simulink model "MtrCtrl_24V"  (R2023b)
settings: Solver=FixedStepDiscrete  StartTime=0.0  StopTime=1  FixedStep=1e-6  RelTol=1e-3
values from neighbouring files (symbols this model uses):
  B = 0.001889    [MtrCtrl_v01.sldd]    (also in PICal.m = 0.001889; PMSM.m = Simulink.Parameter)
  C_LUT_AngleTable_sng_Null = saveVarsMat.C_LUT_AngleTable_sng_Null    [AngleTable.m]    (also in MtrCtrl_v01.sldd = 0.0015339807878856412 0.0030679615757712823 0.00460194236365; PMSM.m; SinLut.m = sinTable(2,:))
  C_LUT_SinTable_sng_Null = saveVarsMat.C_LUT_SinTable_sng_Null    [AngleTable.m]    (also in MtrCtrl_v01.sldd = 0.0015339801862847655 0.0030679567629659761 0.00460192612044; PMSM.m; SinLut.m = sinTable(1,:))
  C_MATH_OneOverSqrtThree_s32n31_Null = 0.57735026918962584    [MtrCtrl_v01.sldd]    (also in PMSM.m = Simulink.Parameter)
  C_MATH_Pi_u32n30_Null = 3.1415926535897931    [MtrCtrl_v01.sldd]    (also in PMSM.m = Simulink.Parameter)
  C_MATH_SqrtThreeOverThree_s32n31_Null = 0.57735026918962573    [MtrCtrl_v01.sldd]    (also in PMSM.m = Simulink.Parameter)
  C_PMSM_CurQKi_u32n31_null = 0.15707963267949    [MtrCtrl_v01.sldd]    (also in PMSM.m = Simulink.Parameter)
  C_PMSM_CurQKp_u32n31_null = 19.949113350295185    [MtrCtrl_v01.sldd]    (also in PMSM.m = Simulink.Parameter)
  C_PMSM_Flux_u32n32_Vs = 0.192    [MtrCtrl_v01.sldd]    (also in PMSM.m = Simulink.Parameter)
  C_PMSM_Ls_pu = 0.398982267005904    [MtrCtrl_v01.sldd]
  C_PMSM_PolePairs_u8_Null = 4.0    [MtrCtrl_v01.sldd]
  Flux = 0.192    [MtrCtrl_v01.sldd]    (also in PICal.m; PMSM.m)
  IBase_A = 2000.0    [MtrCtrl_v01.sldd]    (also in PICal.m = 300; PMSM.m = Simulink.Parameter)
  J = 0.011    [MtrCtrl_v01.sldd]    (also in PICal.m; PMSM.m)
  K_CCM_MRASEna_bool_Flg = 0.0    [MtrCtrl_v01.sldd]
  K_SVM_DefultDuty_s32n31_Null = 0.25    [MtrCtrl_v01.sldd]    (also in PMSM.m = Simulink.Parameter)
  KCCM_VirPosn_flg = 0.0    [MtrCtrl_v01.sldd]    (also in PMSM.m = Simulink.Parameter)
  KCCM_VoltModeEna_Flg = 0.0    [MtrCtrl_v01.sldd]    (also in PMSM.m = Simulink.Parameter)
  Kis = 114583.3333333333    [MtrCtrl_v01.sldd]    (also in PICal.m = 114583.333333; PMSM.m = 114583.333333)
  KSMO_EnaEst_Flg = 0.0    [MtrCtrl_v01.sldd]    (also in PMSM.m = Simulink.Parameter)
  Kt = 1.1520000000000001    [MtrCtrl_v01.sldd]    (also in PICal.m = 1.152; PMSM.m = 1.152)
  Ld = 80e-6    (= 8e-05)    [FluxweakingGen.m]    (also in IEHB_MAPGenerationtest.m = 6.8e-05; MtrCtrl_v01.sldd = 0.000635
                
                    
             ; PICal.m = 0.000635; PMSM.m = Simulink.Parameter)
  LPF_coefg = 0.01    [MtrCtrl_v01.sldd]    (also in PMSM.m = Simulink.Parameter)
  Lq = 80e-6    (= 8e-05)    [FluxweakingGen.m]    (also in IEHB_MAPGenerationtest.m = 6e-05; MtrCtrl_v01.sldd = 0.000685
                
                    
             ; PICal.m = 0.000635; PMSM.m = Simulink.Parameter)
  Ls = 0.000635    [MtrCtrl_v01.sldd]    (also in PICal.m; PMSM.m)
  OneOverUBase_V = 0.0016666666666666668    [MtrCtrl_v01.sldd]    (also in PMSM.m = Simulink.Parameter)
  Pp = 4.0    [MtrCtrl_v01.sldd]    (also in PICal.m = 4; PMSM.m = Simulink.Parameter)
  Rs = 0.03    [FluxweakingGen.m]    (also in MtrCtrl_v01.sldd = 0.05
                
                    
                 ; PICal.m = 0.05; PMSM.m = Simulink.Parameter)
  SecPerRnd = 0.6    [MtrCtrl_v01.sldd]    (also in PMSM.m = Simulink.Parameter)
  sinTable = zeros(2,TableSize)    [SinLut.m]
  SMOGain_V = 323.31615074619043    [MtrCtrl_v01.sldd]    (also in PMSM.m = Simulink.Parameter)
  Ts = 1.0E-6    [MtrCtrl_v01.sldd]    (also in PICal.m = 0.0001; PMSM.m = Simulink.Parameter)
  TsCtrl = 1.0E-6    [MtrCtrl_v01.sldd]
  UBase_V = 600.0    [MtrCtrl_v01.sldd]    (also in PICal.m = 600; PMSM.m = Simulink.Parameter)
  wmBase_rps = 314.15926535897933    [MtrCtrl_v01.sldd]    (also in PICal.m = 314.159265359; PMSM.m = Simulink.Parameter)
undefined symbols (not defined in the file or in its folder): DiscIntNeverNeededParam, Ion, Lithium
libraries: ee_lib x16, spsVoltageMeasurementLib x14, simulink x11, spsSeriesRLCBranchLib x6, spsMosfetLib x6, nesl_utility x6, slpidlib x5, spsCurrentMeasurementLib x4, spsParallelRLCBranchLib x3, simulink_extras x2, spspowerguiLib x2, eePmsmFwController x1
(part 4 of 5)

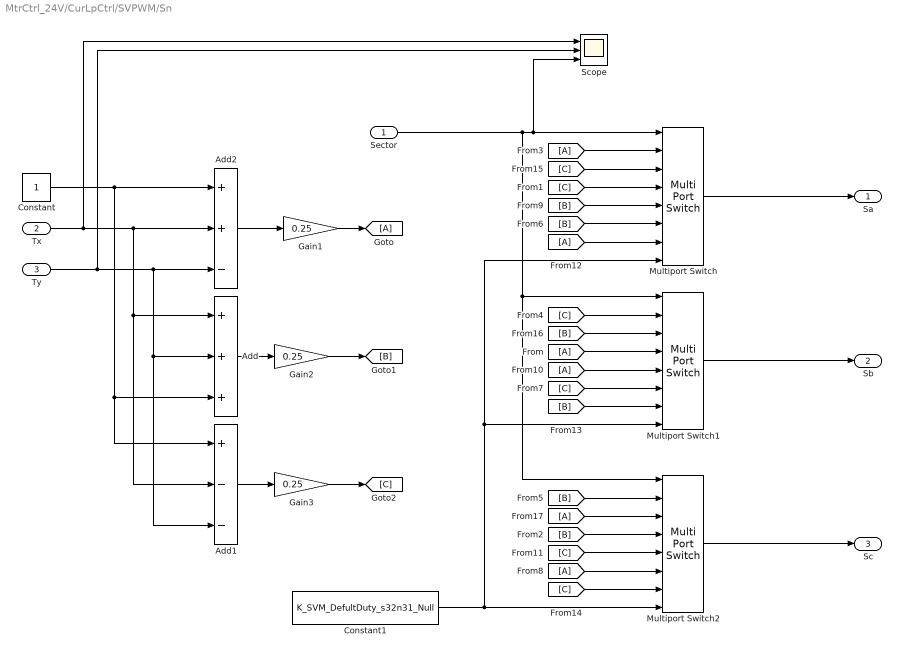
== system MtrCtrl_24V/CurLpCtrl/SVPWM/Sn ==
  Sector : Inport  OutDataTypeStr=uint8
  Tx : Inport  Port=2  OutDataTypeStr=fixdt(0,32,33)
  Ty : Inport  Port=3  OutDataTypeStr=fixdt(0,32,33)
  Add : Sum  Inputs=+++  OutDataTypeStr=fixdt(0,32,31)
  Add1 : Sum  Inputs=+--  OutDataTypeStr=fixdt(0,32,31)
  Add2 : Sum  Inputs=++-  OutDataTypeStr=fixdt(0,32,31)
  Constant : Constant  OutDataTypeStr=fixdt(0,32,31)
  Constant1 : Constant  Value=K_SVM_DefultDuty_s32n31_Null
  From{,3,8,10,12,17} (6 alike) : From
  Gain1 : Gain  Gain=0.25  OutDataTypeStr=fixdt(0,32,33)
  Gain2 : Gain  Gain=0.25  OutDataTypeStr=fixdt(0,32,33)
  Gain3 : Gain  Gain=0.25  OutDataTypeStr=fixdt(0,32,33)
  Goto : Goto
  Multiport Switch : MultiPortSwitch  Inputs=6  DataPortForDefault=Additional data port  OutDataTypeStr=fixdt(0,32,33)  SaturateOnIntegerOverflow=off  InputSameDT=off
  Multiport Switch1 : MultiPortSwitch  Inputs=6  DataPortForDefault=Additional data port  OutDataTypeStr=fixdt(0,32,33)  SaturateOnIntegerOverflow=off  InputSameDT=off
  Multiport Switch2 : MultiPortSwitch  Inputs=6  DataPortForDefault=Additional data port  OutDataTypeStr=fixdt(0,32,33)  SaturateOnIntegerOverflow=off  InputSameDT=off
  Scope : Scope  NumInputPorts=3
  Sa : Outport
  Sb : Outport  Port=2
  Sc : Outport  Port=3
  wires:
  Tx/1 -> Scope/1, Add1/2, Add/1, Add2/2
  Ty/1 -> Scope/2, Add1/3, Add/2, Add2/3
  Add/1 -> Gain2/1
  Constant/1 -> Add1/1, Add/3, Add2/1
  Add2/1 -> Gain1/1
  Add1/1 -> Gain3/1
  Sector/1 -> Multiport Switch/1, Scope/3, Multiport Switch2/1, Multiport Switch1/1
  Multiport Switch/1 -> Sa/1
  Multiport Switch1/1 -> Sb/1
  Multiport Switch2/1 -> Sc/1
  Gain1/1 -> Goto/1
  Gain2/1 -> [B]
  Gain3/1 -> [C]
  [C] -> Multiport Switch/4
  From/1 -> Multiport Switch1/4
  [B] -> Multiport Switch2/4
  From3/1 -> Multiport Switch/2
  [C] -> Multiport Switch1/2
  [B] -> Multiport Switch2/2
  [B] -> Multiport Switch/6
  [C] -> Multiport Switch1/6
  From8/1 -> Multiport Switch2/6
  [B] -> Multiport Switch/5
  From10/1 -> Multiport Switch1/5
  [C] -> Multiport Switch2/5
  From12/1 -> Multiport Switch/7
  [B] -> Multiport Switch1/7
  [C] -> Multiport Switch2/7
  [C] -> Multiport Switch/3
  [B] -> Multiport Switch1/3
  From17/1 -> Multiport Switch2/3
  Constant1/1 -> Multiport Switch/8, Multiport Switch1/8, Multiport Switch2/8

== system MtrCtrl_24V/CurLpCtrl/SVPWM/SwitchTimeCalculation ==
  N : Inport  OutDataTypeStr=fixdt(0,32,29)
  V1 : Inport  Port=2  OutDataTypeStr=fixdt(1,32,31)
  V2 : Inport  Port=3  OutDataTypeStr=fixdt(1,32,32)
  V3 : Inport  Port=4  OutDataTypeStr=fixdt(1,32,32)
  A : MultiPortSwitch  Inputs=6  OutDataTypeStr=fixdt(1,32,32)  SaturateOnIntegerOverflow=off  InputSameDT=off
  B : MultiPortSwitch  Inputs=6  OutDataTypeStr=fixdt(1,32,31)  SaturateOnIntegerOverflow=off  InputSameDT=off
  C : MultiPortSwitch  Inputs=6  OutDataTypeStr=fixdt(1,32,31)  SaturateOnIntegerOverflow=off  InputSameDT=off
  Gain1 : Gain  Gain=-1  ParamDataTypeStr=fixdt(1,32,31)  OutDataTypeStr=fixdt(1,32,32)
  Gain2 : Gain  Gain=-1  ParamDataTypeStr=fixdt(1,32,31)  OutDataTypeStr=fixdt(1,32,31)
  Gain3 : Gain  Gain=-1  ParamDataTypeStr=fixdt(1,32,31)  OutDataTypeStr=fixdt(1,32,32)
  Sum : Sum  Inputs=|++  OutDataTypeStr=fixdt(1,32,32)  AccumDataTypeStr=fixdt(1,32,32)
  Sum1 : Sum  Inputs=-+|  OutDataTypeStr=fixdt(1,32,30)  AccumDataTypeStr=fixdt(1,32,30)
  Sum2 : Sum  Inputs=|++  OutDataTypeStr=fixdt(1,32,30)  AccumDataTypeStr=fixdt(1,32,30)
  Ta : Outport
  Tb : Outport  Port=2
  Tc : Outport  Port=3
  wires:
  N/1 -> A/1, B/1, C/1
  A/1 -> Ta/1
  B/1 -> Tb/1
  C/1 -> Tc/1
  V2/1 -> Gain1/1, A/2, A/5, Sum/1
  V3/1 -> Gain3/1, A/7, A/4, Sum/2, Sum1/1
  Sum/1 -> A/6, A/3
  V1/1 -> Gain2/1, B/3, B/6, Sum1/2
  Sum1/1 -> B/2, B/5
  Gain3/1 -> B/4, B/7
  Gain1/1 -> C/5, C/2, Sum2/1
  Gain2/1 -> C/3, C/6, Sum2/2
  Sum2/1 -> C/7, C/4

== system MtrCtrl_24V/CurLpCtrl/SVPWM/TempValueCalculation ==
  V_alpha : Inport  OutDataTypeStr=fixdt(1,32,31)
  V_beta : Inport  Port=2  OutDataTypeStr=fixdt(1,32,31)
  Add : Sum  Inputs=+-  OutDataTypeStr=fixdt(1,32,32)
  Add1 : Sum  OutDataTypeStr=fixdt(1,32,32)
  Gain : Gain  Gain=0.5  OutDataTypeStr=fixdt(1,32,32)
  Gain1 : Gain  Gain=sqrt(3)/2  OutDataTypeStr=fixdt(1,32,33)
  V1 : Outport  VectorParamsAs1DForOutWhenUnconnected=off
  V2 : Outport  Port=2  VectorParamsAs1DForOutWhenUnconnected=off
  V3 : Outport  Port=3  VectorParamsAs1DForOutWhenUnconnected=off
  wires:
  V_alpha/1 -> Gain1/1
  Gain1/1 -> Add1/2
  Add1/1 -> V2/1, Add/1  "V2"
  V_beta/1 -> Gain/1, Add/2, V1/1  "V1"
  Add/1 -> V3/1  "V3"
  Gain/1 -> Add1/1

== system MtrCtrl_24V/CurLpCtrl/Subsystem10/Subsystem ==
  idqRef : Inport  OutDataTypeStr=fixdt(1,32,31)
  vdq : Inport  Port=2  OutDataTypeStr=fixdt(1,32,31)
  VphMax : Inport  Port=3  OutDataTypeStr=fixdt(0,32,32)
  Cartesian to Polar : Subsystem  Tag=DecoupledSystem
  Constant : Constant  Value=C_MATH_Pi_u32n30_Null  OutDataTypeStr=fixdt(0,32,30)  SampleTime=-1
  Demux : Demux  Outputs=2
  Discrete-Time Integrator : DiscreteIntegrator  IntegratorMethod=Integration: Backward Euler  gainval=5  InitialCondition=1  SampleTime=-1  OutDataTypeStr=fixdt(1,32,28)  ICPrevOutput=DiscIntNeverNeededParam  ICPrevScaledInput=DiscIntNeverNeededParam
  Gain : Gain  Gain=50  OutDataTypeStr=fixdt(1,32,25)
  Gain1 : Gain  Gain=10  OutDataTypeStr=fixdt(1,32,25)
  Gain2 : Gain  Gain=2
  Modulation index threshold : Constant  Value=C_MATH_SqrtThreeOverThree_s32n31_Null  OutDataTypeStr=fixdt(0,32,31)  SampleTime=-1
  Modulation index threshold1 : Constant  Value=3.24  OutDataTypeStr=fixdt(0,32,30)  SampleTime=-1
  Mux : Mux  Inputs=2
  Polar to Cartesian : Subsystem  Tag=DecoupledSystem
  Product : Product  OutDataTypeStr=fixdt(1,32,28)
  Saturation : Saturate  UpperLimit=1  LowerLimit=0  OutDataTypeStr=fixdt(1,32,28)
  Subsystem1 : Subsystem
  Sum : Sum  Inputs=|-+  OutDataTypeStr=fixdt(1,32,30)
  Sum1 : Sum  Inputs=|-+  OutDataTypeStr=fixdt(1,32,28)
  Sum2 : Sum  Inputs=|-+  OutDataTypeStr=fixdt(1,32,28)
  Sum3 : Sum  Inputs=-+  OutDataTypeStr=fixdt(1,32,28)
  Sum4 : Sum  Inputs=|++  OutDataTypeStr=fixdt(1,32,25)
  Unit Delay : UnitDelay  SampleTime=-1  HasFrameUpgradeWarning=on
  idqRefFW : Outport  VectorParamsAs1DForOutWhenUnconnected=off
  wires:
  Product/1 -> Sum2/1
  Sum1/1 -> Product/1
  Gain1/1 -> Sum4/2
  Cartesian to Polar/1(Out1) -> Polar to Cartesian/1(In1)
  Subsystem1/1(M) -> Sum/1
  Sum/1 -> Gain/1
  Discrete-Time Integrator/1 -> Saturation/1, Sum3/1
  Unit Delay/1 -> Gain1/1
  Cartesian to Polar/2(Out2) -> Sum1/1
  Polar to Cartesian/2(Out2) -> Mux/2
  Mux/1 -> idqRefFW/1
  Gain/1 -> Sum4/1
  VphMax/1 -> Subsystem1/2(VphMax)
  Modulation index threshold/1 -> Gain2/1
  Saturation/1 -> Product/2, Sum3/2
  Demux/2 -> Cartesian to Polar/2(In2)
  Demux/1 -> Cartesian to Polar/1(In1)
  idqRef/1 -> Demux/1
  Polar to Cartesian/1(Out1) -> Mux/1
  Constant/1 -> Sum1/2, Sum2/2
  Sum3/1 -> Unit Delay/1
  vdq/1 -> Subsystem1/1(vdq)
  Sum2/1 -> Polar to Cartesian/2(In2)
  Sum4/1 -> Discrete-Time Integrator/1
  Gain2/1 -> Sum/2

== system MtrCtrl_24V/CurLpCtrl/Subsystem2/Subsystem1 ==
  In1 : Inport  OutDataTypeStr=fixdt(0,32,0)
  Constant7 : Constant  Value=2*pi  OutDataTypeStr=fixdt(0,32,0)
  Mod : Math  Operator=mod
  Out1 : Outport
  wires:
  Mod/1 -> Out1/1
  In1/1 -> Mod/1
  Constant7/1 -> Mod/2

== system MtrCtrl_24V/CurLpCtrl/Subsystem2/Subsystem2 ==
  FilterIn : Inport  OutDataTypeStr=fixdt(1,32,31)
  Rest : Inport  Port=2  OutDataTypeStr=fixdt(1,32,0)
  Add : Sum  Inputs=+-  OutDataTypeStr=fixdt(1,32,31)
  Add1 : Sum  OutDataTypeStr=fixdt(1,32,31)
  Constant : Constant  Value=LPF_coefg  OutDataTypeStr=fixdt(0,32,31)
  Delay : Delay  DelayLength=1  ExternalReset=Either
      settings: InputPortMap=u0,r5
  Product : Product  OutDataTypeStr=fixdt(1,32,31)
  FilterOut : Outport
  wires:
  FilterIn/1 -> Add/1
  Add/1 -> Product/2
  Product/1 -> Add1/1
  Add1/1 -> Delay/1, FilterOut/1
  Delay/1 -> Add/2, Add1/2
  Rest/1 -> Delay/2
  Constant/1 -> Product/1

== system MtrCtrl_24V/CurLpCtrl/Subsystem2/Subsystem3 ==
  ParkPosn : Inport  OutDataTypeStr=fixdt(1,32,28)
  1-D Lookup Table : Lookup_n-D  NumberOfTableDimensions=1  BreakpointsForDimension1=sinTable(2,:)  BeginIndexSearchUsingPreviousIndexResult=on  Table=sinTable(1,:)  ExtrapMethod=Clip  UseLastTableValue=on  ApplyFullPrecisionForLinearInterpolation=on  InternalRulePriority=Speed  OutDataTypeStr=fixdt(0,32,31)  RndMeth=Simplest
  1-D Lookup Table1 : Lookup_n-D  NumberOfTableDimensions=1  BreakpointsForDimension1=sinTable(2,:)  BeginIndexSearchUsingPreviousIndexResult=on  Table=sinTable(1,:)  ExtrapMethod=Clip  UseLastTableValue=on  ApplyFullPrecisionForLinearInterpolation=on  InternalRulePriority=Speed  OutDataTypeStr=fixdt(0,32,31)  RndMeth=Simplest
  Add : Sum  OutDataTypeStr=fixdt(1,32,26)
  Chart : Stateflow chart  TreatAsAtomicUnit=on
  Constant1 : Constant  Value=0  OutDataTypeStr=fixdt(1,32,4)
  Gain : Gain  Gain=4  OutDataTypeStr=fixdt(1,32,26)
  Product : Product  OutDataTypeStr=fixdt(1,32,30)  RndMeth=Simplest
  Product1 : Product  OutDataTypeStr=fixdt(1,32,30)
  Scope : Scope  NumInputPorts=3
  SinTheta : Outport
  CosTheta : Outport  Port=2
  wires:
  ParkPosn/1 -> Gain/1
  Gain/1 -> Add/2
  Constant1/1 -> Add/1
  Product/1 -> Scope/1, SinTheta/1
  Product1/1 -> Scope/2, CosTheta/1
  Add/1 -> Scope/3, Chart/1(Angle)
  Chart/1(SinAngle) -> 1-D Lookup Table/1
  Chart/3(CosAngle) -> 1-D Lookup Table1/1
  1-D Lookup Table/1 -> Product/1
  Chart/2(SinSign) -> Product/2
  1-D Lookup Table1/1 -> Product1/1
  Chart/4(CosSign) -> Product1/2

== system MtrCtrl_24V/CurLpCtrl/Subsystem2/Subsystem4 ==
  FilterIn : Inport  OutDataTypeStr=fixdt(1,32,31)
  Rest : Inport  Port=2  OutDataTypeStr=fixdt(1,32,0)
  Add : Sum  Inputs=+-  OutDataTypeStr=fixdt(1,32,31)
  Add1 : Sum  OutDataTypeStr=fixdt(1,32,31)
  Constant : Constant  Value=LPF_coefg  OutDataTypeStr=fixdt(0,32,31)
  Delay : Delay  DelayLength=1  ExternalReset=Either
      settings: InputPortMap=u0,r5
  Product : Product  OutDataTypeStr=fixdt(1,32,31)
  FilterOut : Outport
  wires:
  Rest/1 -> Delay/2
  Delay/1 -> Add1/2, Add/2
  Add1/1 -> FilterOut/1, Delay/1
  Product/1 -> Add1/1
  Add/1 -> Product/2
  FilterIn/1 -> Add/1
  Constant/1 -> Product/1

== system MtrCtrl_24V/CurLpCtrl/Subsystem2/Subsystem5 ==
  FilterIn : Inport  OutDataTypeStr=fixdt(1,32,22)
  Rest : Inport  Port=2  OutDataTypeStr=fixdt(1,32,0)
  Add : Sum  Inputs=+-  OutDataTypeStr=fixdt(1,32,23)
  Add1 : Sum  OutDataTypeStr=fixdt(1,32,22)
  Constant : Constant  Value=LPF_coefg  OutDataTypeStr=fixdt(0,32,38)
  Delay : Delay  DelayLength=1  ExternalReset=Either
      settings: InputPortMap=u0,r5
  Product : Product  OutDataTypeStr=fixdt(1,32,29)
  FilterOut : Outport
  wires:
  FilterIn/1 -> Add/1
  Add/1 -> Product/2
  Product/1 -> Add1/1
  Add1/1 -> Delay/1, FilterOut/1
  Delay/1 -> Add/2, Add1/2
  Rest/1 -> Delay/2
  Constant/1 -> Product/1

== system MtrCtrl_24V/CurLpCtrl/Subsystem2/Z_alpha ==
  Salpha : Inport  OutDataTypeStr=int32
  Constant : Constant  OutDataTypeStr=fixdt(1,32,30)
  Constant1 : Constant  Value=-1  OutDataTypeStr=fixdt(1,32,30)
  Divide : Product  Inputs=*/  OutDataTypeStr=fixdt(1,32,30)
  E : Constant  Value=600  OutDataTypeStr=int32
  If : If  NumInputs=2  IfExpression=u1 > u2  ElseIfExpressions=u1 < -u2
  If Action Subsystem : Subsystem  TreatAsAtomicUnit=on
  If Action Subsystem1 : Subsystem  TreatAsAtomicUnit=on
  If Action Subsystem2 : Subsystem  TreatAsAtomicUnit=on
  Merge : Merge  Inputs=3
  ZalphaOut : Outport
  wires:
  Salpha/1 -> If/1, Divide/1
  E/1 -> If/2, Divide/2
  Divide/1 -> If Action Subsystem2/1(In1)
  If/1 -> If Action Subsystem/Action
  If Action Subsystem/1(ZalphaOut) -> Merge/1
  If/3 -> If Action Subsystem2/Action
  If/2 -> If Action Subsystem1/Action
  If Action Subsystem1/1(ZalphaOut) -> Merge/2
  If Action Subsystem2/1(ZalphaOut) -> Merge/3
  Merge/1 -> ZalphaOut/1
  Constant/1 -> If Action Subsystem/1(In1)
  Constant1/1 -> If Action Subsystem1/1(In1)

== system MtrCtrl_24V/CurLpCtrl/Subsystem2/Z_alpha1 ==
  Salpha : Inport  OutDataTypeStr=int32
  Constant : Constant  OutDataTypeStr=fixdt(1,32,30)
  Constant1 : Constant  Value=-1  OutDataTypeStr=fixdt(1,32,30)
  Divide : Product  Inputs=*/  OutDataTypeStr=fixdt(1,32,30)
  E : Constant  Value=600  OutDataTypeStr=int32
  If : If  NumInputs=2  IfExpression=u1 > u2  ElseIfExpressions=u1 < -u2
  If Action Subsystem : Subsystem  TreatAsAtomicUnit=on
  If Action Subsystem1 : Subsystem  TreatAsAtomicUnit=on
  If Action Subsystem2 : Subsystem  TreatAsAtomicUnit=on
  Merge : Merge  Inputs=3
  ZalphaOut : Outport
  wires:
  Constant1/1 -> If Action Subsystem1/1(In1)
  Constant/1 -> If Action Subsystem/1(In1)
  Merge/1 -> ZalphaOut/1
  If Action Subsystem2/1(ZalphaOut) -> Merge/3
  If Action Subsystem1/1(ZalphaOut) -> Merge/2
  If/2 -> If Action Subsystem1/Action
  If/3 -> If Action Subsystem2/Action
  If Action Subsystem/1(ZalphaOut) -> Merge/1
  If/1 -> If Action Subsystem/Action
  Divide/1 -> If Action Subsystem2/1(In1)
  E/1 -> Divide/2, If/2
  Salpha/1 -> Divide/1, If/1

== system MtrCtrl_24V/CurLpCtrl/Subsystem4/SinCos ==
  In1 : Inport  LockScale=on
  DTC_input_1 : DataTypeConversion  OutDataTypeStr=fixdt('double')  RndMeth=Nearest  SaturateOnIntegerOverflow=off  LockScale=on
  DTC_output_1 : DataTypeConversion  OutDataTypeStr=fixdt(1,32,4)  SaturateOnIntegerOverflow=off  RndMeth=Floor
  DTC_output_2 : DataTypeConversion  OutDataTypeStr=fixdt(0,32,31)  SaturateOnIntegerOverflow=off  RndMeth=Floor
  ReplicaOfSource : Trigonometry  Operator=sincos
  Out1 : Outport  LockScale=on
  Out2 : Outport  Port=2  LockScale=on
  wires:
  In1/1 -> DTC_input_1/1
  DTC_output_1/1 -> Out1/1
  ReplicaOfSource/1 -> DTC_output_1/1
  ReplicaOfSource/2 -> DTC_output_2/1
  DTC_input_1/1 -> ReplicaOfSource/1
  DTC_output_2/1 -> Out2/1

== system MtrCtrl_24V/CurLpCtrl/Subsystem8/Subsystem ==
  Id_k : Inport
  Iq_k : Inport  Port=2
  we_k : Inport  Port=3
  Ud_k : Inport  Port=4
  Uq_k : Inport  Port=5
  Add2 : Sum
  Add3 : Sum
  Add4 : Sum
  Add5 : Sum  Inputs=+++
  Constant1 : Constant  Value=1-TsCtrl*Rs/Ls
  Constant18 : Constant  Value=-TsCtrl*Flux/Ls
  Constant2 : Constant  Value=TsCtrl/Ls
  Constant3 : Constant  Value=1-TsCtrl*Rs/Ls
  Constant4 : Constant  Value=TsCtrl/Ls
  Gain6 : Gain  Gain=TsCtrl
  Gain7 : Gain  Gain=-1
  Id_k_copy : InportShadow
  Iq_k_copy : InportShadow  Port=2
  Product{5,9..14} (7 alike) : Product
  Subtract : Sum  Inputs=+-
  Subtract1 : Sum  Inputs=+-
  Dlt_Id : Outport
  Dlt_Iq : Outport  Port=2
  wires:
  Product14/1 -> Add5/3
  Constant2/1 -> Product13/1
  Product10/1 -> Add3/1
  Gain6/1 -> Gain7/1, Product9/2
  Constant1/1 -> Product11/1
  Uq_k/1 -> Product13/2
  Product5/1 -> Add2/1
  Product9/1 -> Add2/2
  Product12/1 -> Add4/2
  Id_k/1 -> Product10/2, Product5/1
  Product11/1 -> Add3/2
  Constant4/1 -> Product12/1
  Add2/1 -> Add4/1
  Iq_k/1 -> Product11/2, Product9/1
  Constant18/1 -> Product14/1
  Add5/1 -> Subtract1/1  "Iq_k_1"
  we_k/1 -> Product14/2, Gain6/1
  Gain7/1 -> Product10/1
  Constant3/1 -> Product5/2
  Add3/1 -> Add5/1
  Add4/1 -> Subtract/1  "Id_k_1"
  Product13/1 -> Add5/2
  Ud_k/1 -> Product12/2
  Id_k_copy/1 -> Subtract/2
  Subtract/1 -> Dlt_Id/1
  Subtract1/1 -> Dlt_Iq/1
  Iq_k_copy/1 -> Subtract1/2

== system MtrCtrl_24V/CurLpCtrl/Subsystem8/Subsystem3 ==
  Id_k1 : Inport
  Iq_k1 : Inport  Port=2
  we_k : Inport  Port=3
  Ud_k1 : Inport  Port=4
  Uq_k1 : Inport  Port=5
  Add2 : Sum
  Add3 : Sum
  Add4 : Sum
  Add5 : Sum  Inputs=+++
  Constant1 : Constant  Value=1-Ts*Rs/Ls
  Constant14 : Constant  Value=1-Ts*Rs/Ls
  Constant16 : Constant  Value=Ts/Ls
  Constant18 : Constant  Value=-Ts*Flux/Ls
  Constant2 : Constant  Value=Ts/Ls
  Gain6 : Gain  Gain=TsCtrl
  Gain7 : Gain  Gain=-1
  Id_k1_Copy : InportShadow
  Iq_k1_Copy : InportShadow  Port=2
  Product{5,9..14} (7 alike) : Product
  Subtract : Sum  Inputs=+-
  Subtract1 : Sum  Inputs=+-
  Dlt_Id : Outport
  Dlt_Iq : Outport  Port=2
  wires:
  Iq_k1_Copy/1 -> Subtract1/2
  Subtract1/1 -> Dlt_Iq/1
  Subtract/1 -> Dlt_Id/1
  Id_k1_Copy/1 -> Subtract/2
  Ud_k1/1 -> Product12/2
  Product13/1 -> Add5/2
  Add4/1 -> Subtract/1  "Id_k2"
  Add3/1 -> Add5/1
  Constant14/1 -> Product5/2
  Gain7/1 -> Product10/1
  we_k/1 -> Gain6/1, Product14/2
  Add5/1 -> Subtract1/1  "Iq_k2"
  Constant18/1 -> Product14/1
  Iq_k1/1 -> Product9/1, Product11/2
  Add2/1 -> Add4/1
  Constant16/1 -> Product12/1
  Product11/1 -> Add3/2
  Id_k1/1 -> Product5/1, Product10/2
  Product12/1 -> Add4/2
  Product9/1 -> Add2/2
  Product5/1 -> Add2/1
  Uq_k1/1 -> Product13/2
  Constant1/1 -> Product11/1
  Gain6/1 -> Product9/2, Gain7/1
  Product10/1 -> Add3/1
  Constant2/1 -> Product13/1
  Product14/1 -> Add5/3

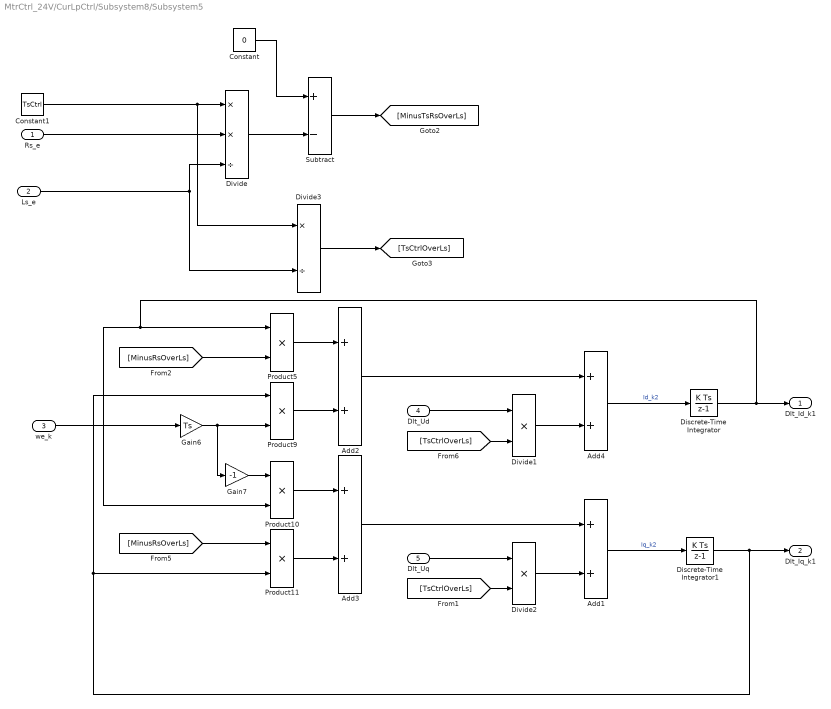
== system MtrCtrl_24V/CurLpCtrl/Subsystem8/Subsystem5 ==
  Rs_e : Inport
  Ls_e : Inport  Port=2
  we_k : Inport  Port=3
  Dlt_Ud : Inport  Port=4
  Dlt_Uq : Inport  Port=5
  Add{1..4} (4 alike) : Sum
  Constant : Constant  Value=0
  Constant1 : Constant  Value=TsCtrl
  Discrete-Time Integrator : DiscreteIntegrator  SampleTime=-1  ICPrevOutput=DiscIntNeverNeededParam  ICPrevScaledInput=DiscIntNeverNeededParam
  Discrete-Time Integrator1 : DiscreteIntegrator  SampleTime=-1  ICPrevOutput=DiscIntNeverNeededParam  ICPrevScaledInput=DiscIntNeverNeededParam
  Divide : Product  Inputs=**/
  Divide1 : Product  Inputs=**
  Divide2 : Product  Inputs=**
  Divide3 : Product  Inputs=*/
  Gain6 : Gain  Gain=Ts
  Gain7 : Gain  Gain=-1
  Product{5,9..11} (4 alike) : Product
  Subtract : Sum  Inputs=+-
  Dlt_Id_k1 : Outport
  Dlt_Iq_k1 : Outport  Port=2
  wires:
  Dlt_Ud/1 -> Divide1/1
  Divide2/1 -> Add1/2
  Add4/1 -> Discrete-Time Integrator/1  "Id_k2"
  Add3/1 -> Add1/1
  [MinusRsOverLs] -> Product5/2
  Gain7/1 -> Product10/1
  we_k/1 -> Gain6/1
  Add1/1 -> Discrete-Time Integrator1/1  "Iq_k2"
  Discrete-Time Integrator1/1 -> Dlt_Iq_k1/1, Product9/1, Product11/2
  Add2/1 -> Add4/1
  [TsCtrlOverLs] -> Divide1/2
  Product11/1 -> Add3/2
  Discrete-Time Integrator/1 -> Product10/2, Product5/1, Dlt_Id_k1/1
  Divide1/1 -> Add4/2
  Product9/1 -> Add2/2
  Product5/1 -> Add2/1
  Dlt_Uq/1 -> Divide2/1
  [MinusRsOverLs] -> Product11/1
  Gain6/1 -> Product9/2, Gain7/1
  Product10/1 -> Add3/1
  Constant/1 -> Subtract/1
  Rs_e/1 -> Divide/2
  Divide/1 -> Subtract/2
  Subtract/1 -> [MinusTsRsOverLs]
  Ls_e/1 -> Divide3/2, Divide/3
  [TsCtrlOverLs] -> Divide2/2
  Constant1/1 -> Divide3/1, Divide/1
  Divide3/1 -> [TsCtrlOverLs]

== system MtrCtrl_24V/CurLpCtrl/Subsystem8/Subsystem6 ==
  Id : Inport
  Iq : Inport  Port=2
  Id_e : Inport  Port=3
  Iq_e : Inport  Port=4
  Abs : Abs  SaturateOnIntegerOverflow=off
  Add : Sum
  Constant2 : Constant
  Constant3 : Constant  Value=0.2
  Constant8 : Constant  Commented=on  Value=2*Rs/Ls
  PID Controller : slpidlib/PID Controller  Controller=PI  Form=Parallel  TimeDomain=Discrete-time  UseExternalTs=off  SampleTime=-1  IntegratorMethod=Forward Euler  FilterMethod=Forward Euler  ControllerParametersSource=external  P=1  I=1  UseKiTs=off  D=0  N=100  UseFilter=on  TunerSelectOption=Transfer Function Based (PID Tuner App)  InitialConditionSource=internal  InitialConditionForIntegrator=0  InitialConditionForFilter=0  DifferentiatorICPrevScaledInput=0  ExternalReset=none  TrackingMode=off  Kt=1  LimitOutput=off  SatLimitsSource=internal  UpperSaturationLimit=inf  LowerSaturationLimit=-inf  LinearizeAsGain=on  AntiWindupMode=none  Kb=1  LimitIntegrator=off  UpperIntegratorSaturationLimit=inf  LowerIntegratorSaturationLimit=-inf  POutMin=[]  POutMax=[]  IOutMin=[]  IOutMax=[]  DOutMin=[]  DOutMax=[]  NOutMin=[]  NOutMax=[]  SumOutMin=[]  SumOutMax=[]  SaturationOutMin=[]  SaturationOutMax=[]  PParamMin=[]  PParamMax=[]  IParamMin=[]  IParamMax=[]  DParamMin=[]  DParamMax=[]  NParamMin=[]  NParamMax=[]  KbParamMin=[]  KbParamMax=[]  KtParamMin=[]  KtParamMax=[]  KbOutMin=[]  KbOutMax=[]  KtOutMin=[]  KtOutMax=[]  IntegratorOutMin=[]  IntegratorOutMax=[]  FilterOutMin=[]  FilterOutMax=[]  SumI1OutMin=[]  SumI1OutMax=[]  SumI2OutMin=[]  SumI2OutMax=[]  SumI3OutMin=[]  SumI3OutMax=[]  SumI4OutMin=[]  SumI4OutMax=[]  SumDOutMin=[]  SumDOutMax=[]  DifferentiatorOutMin=[]  DifferentiatorOutMax=[]  FilterDiffOutCoefMin=[]  FilterDiffOutCoefMax=[]  ReciprocalOutMin=[]  ReciprocalOutMax=[]  SumDenOutMin=[]  SumDenOutMax=[]  SumNumOutMin=[]  SumNumOutMax=[]  DivideOutMin=[]  DivideOutMax=[]  UdiffTsProdOutMin=[]  UdiffTsProdOutMax=[]  NTsProdOutMin=[]  NTsProdOutMax=[]  UintegralTsProdOutMin=[]  UintegralTsProdOutMax=[]  UngainTsProdOutMin=[]  UngainTsProdOutMax=[]  ClampingZeroOutDataTypeStr=Inherit: Inherit via back propagation  ClampingZeroOutMin=[]  ClampingZeroOutMax=[]  FilterDenConstantOutDataTypeStr=Inherit: Inherit via back propagation  FilterDenConstantOutMin=[]  FilterDenConstantOutMax=[]  PCopyOutDataTypeStr=Inherit: Inherit via back propagation  PCopyOutMin=[]  PCopyOutMax=[]  NCopyOutDataTypeStr=Inherit: Inherit via back propagation  NCopyOutMin=[]  NCopyOutMax=[]  IntegratorContinuousStateAttributes=''  IntegratorStateMustResolveToSignalObject=off  IntegratorRTWStateStorageClass=Auto  FilterContinuousStateAttributes=''  FilterStateMustResolveToSignalObject=off  FilterRTWStateStorageClass=Auto  ParallelPVariant=ExternalParameters  IdealPVariant=Disabled  IVariant=ExternalParameters  DVariant=Disabled  IntegratorVariant=Discrete  SatVariant=Disabled  AWVariant=Passthrough  PCopyVariant=Disabled  TRVariant=Disabled  FdbkBlocksVariant=Forward  IdealPFdbkVariant=Disabled  SatFdbkVariant=Disabled  DerivativeFilterVariant=Disabled  NVariant=Disabled  NCopyVariant=Disabled_SignalSpec  FilterICVariant=Disabled  IntegratorICVariant=InternalICs  ExternalResetVariant=Disabled  TRSumVariant=Passthrough  SumFdbkVariant=Disabled  SumVariant=Sum_PI  TsampFilterVariant=InternalTs  TsampNgainVariant=Passthrough  TsampIntegralVariant=Disabled_SignalSpec  ExternalSaturationOutDataTypeStr=Inherit: Same as second input
  Product3 : Product
  Product5 : Product
  Saturation : Saturate  UpperLimit=20*Rs/Ls  LowerLimit=1e-6
  Subtract6 : Sum  Inputs=+-
  Subtract7 : Sum  Inputs=+-
  PIOut : Outport
  wires:
  Iq/1 -> Subtract7/1
  Id/1 -> Subtract6/1
  Constant8/1 -> ?
  Product3/1 -> Add/1
  Subtract6/1 -> Product3/1
  Product5/1 -> Add/2
  Iq_e/1 -> Subtract7/2, Product5/2
  Subtract7/1 -> Product5/1
  Id_e/1 -> Product3/2, Subtract6/2
  PID Controller/1 -> Saturation/1
  Constant2/1 -> PID Controller/2
  Abs/1 -> PID Controller/1
  Constant3/1 -> PID Controller/3
  Saturation/1 -> PIOut/1
  Add/1 -> Abs/1

== system MtrCtrl_24V/CurLpCtrl/Subsystem8/Subsystem7 ==
  Id : Inport
  Iq : Inport  Port=2
  Id_e : Inport  Port=3
  Iq_e : Inport  Port=4
  Ud : Inport  Port=5
  Uq : Inport  Port=6
  Abs : Abs  SaturateOnIntegerOverflow=off
  Add : Sum
  Constant2 : Constant
  Constant3 : Constant  Value=0.2
  Constant8 : Constant  Commented=on  Value=1/2/Ls
  Delay : Delay  DelayLength=1
  Delay1 : Delay  DelayLength=1
  PID Controller : slpidlib/PID Controller  Controller=PI  Form=Parallel  TimeDomain=Discrete-time  UseExternalTs=off  SampleTime=-1  IntegratorMethod=Forward Euler  FilterMethod=Forward Euler  ControllerParametersSource=external  P=1  I=1  UseKiTs=off  D=0  N=100  UseFilter=on  TunerSelectOption=Transfer Function Based (PID Tuner App)  InitialConditionSource=internal  InitialConditionForIntegrator=0  InitialConditionForFilter=0  DifferentiatorICPrevScaledInput=0  ExternalReset=none  TrackingMode=off  Kt=1  LimitOutput=off  SatLimitsSource=internal  UpperSaturationLimit=inf  LowerSaturationLimit=-inf  LinearizeAsGain=on  AntiWindupMode=none  Kb=1  LimitIntegrator=off  UpperIntegratorSaturationLimit=inf  LowerIntegratorSaturationLimit=-inf  POutMin=[]  POutMax=[]  IOutMin=[]  IOutMax=[]  DOutMin=[]  DOutMax=[]  NOutMin=[]  NOutMax=[]  SumOutMin=[]  SumOutMax=[]  SaturationOutMin=[]  SaturationOutMax=[]  PParamMin=[]  PParamMax=[]  IParamMin=[]  IParamMax=[]  DParamMin=[]  DParamMax=[]  NParamMin=[]  NParamMax=[]  KbParamMin=[]  KbParamMax=[]  KtParamMin=[]  KtParamMax=[]  KbOutMin=[]  KbOutMax=[]  KtOutMin=[]  KtOutMax=[]  IntegratorOutMin=[]  IntegratorOutMax=[]  FilterOutMin=[]  FilterOutMax=[]  SumI1OutMin=[]  SumI1OutMax=[]  SumI2OutMin=[]  SumI2OutMax=[]  SumI3OutMin=[]  SumI3OutMax=[]  SumI4OutMin=[]  SumI4OutMax=[]  SumDOutMin=[]  SumDOutMax=[]  DifferentiatorOutMin=[]  DifferentiatorOutMax=[]  FilterDiffOutCoefMin=[]  FilterDiffOutCoefMax=[]  ReciprocalOutMin=[]  ReciprocalOutMax=[]  SumDenOutMin=[]  SumDenOutMax=[]  SumNumOutMin=[]  SumNumOutMax=[]  DivideOutMin=[]  DivideOutMax=[]  UdiffTsProdOutMin=[]  UdiffTsProdOutMax=[]  NTsProdOutMin=[]  NTsProdOutMax=[]  UintegralTsProdOutMin=[]  UintegralTsProdOutMax=[]  UngainTsProdOutMin=[]  UngainTsProdOutMax=[]  ClampingZeroOutDataTypeStr=Inherit: Inherit via back propagation  ClampingZeroOutMin=[]  ClampingZeroOutMax=[]  FilterDenConstantOutDataTypeStr=Inherit: Inherit via back propagation  FilterDenConstantOutMin=[]  FilterDenConstantOutMax=[]  PCopyOutDataTypeStr=Inherit: Inherit via back propagation  PCopyOutMin=[]  PCopyOutMax=[]  NCopyOutDataTypeStr=Inherit: Inherit via back propagation  NCopyOutMin=[]  NCopyOutMax=[]  IntegratorContinuousStateAttributes=''  IntegratorStateMustResolveToSignalObject=off  IntegratorRTWStateStorageClass=Auto  FilterContinuousStateAttributes=''  FilterStateMustResolveToSignalObject=off  FilterRTWStateStorageClass=Auto  ParallelPVariant=ExternalParameters  IdealPVariant=Disabled  IVariant=ExternalParameters  DVariant=Disabled  IntegratorVariant=Discrete  SatVariant=Disabled  AWVariant=Passthrough  PCopyVariant=Disabled  TRVariant=Disabled  FdbkBlocksVariant=Forward  IdealPFdbkVariant=Disabled  SatFdbkVariant=Disabled  DerivativeFilterVariant=Disabled  NVariant=Disabled  NCopyVariant=Disabled_SignalSpec  FilterICVariant=Disabled  IntegratorICVariant=InternalICs  ExternalResetVariant=Disabled  TRSumVariant=Passthrough  SumFdbkVariant=Disabled  SumVariant=Sum_PI  TsampFilterVariant=InternalTs  TsampNgainVariant=Passthrough  TsampIntegralVariant=Disabled_SignalSpec  ExternalSaturationOutDataTypeStr=Inherit: Same as second input
  Product3 : Product
  Product5 : Product
  Saturation1 : Saturate  UpperLimit=1e6  LowerLimit=0.1
  Scope : Scope
  Subtract{1..2,6..7} (4 alike) : Sum  Inputs=+-
  PIOut : Outport
  wires:
  Id_e/1 -> Subtract6/2
  Add/1 -> Abs/1
  Subtract7/1 -> Product5/1
  Iq_e/1 -> Subtract7/2
  Product5/1 -> Add/2
  Subtract6/1 -> Product3/1
  Product3/1 -> Add/1
  Constant8/1 -> ?
  Id/1 -> Subtract6/1
  PID Controller/1 -> Scope/1, Saturation1/1
  Iq/1 -> Subtract7/1
  Delay/1 -> Subtract1/2
  Ud/1 -> Delay/1, Subtract1/1
  Subtract1/1 -> Product3/2
  Delay1/1 -> Subtract2/2
  Uq/1 -> Delay1/1, Subtract2/1
  Subtract2/1 -> Product5/2
  Saturation1/1 -> PIOut/1
  Constant3/1 -> PID Controller/3
  Abs/1 -> PID Controller/1
  Constant2/1 -> PID Controller/2

== system MtrCtrl_24V/Inverter/Subsystem/Subsystem1 ==
  CaptureEna : Inport
  Add : Sum
  Constant : Constant  Value=2.5
  Constant1 : Constant  Value=5
  Constant2 : Constant  Value=4096
  Constant3 : Constant  Value=2048
  Constant4 : Constant  Value=0.2442
  Divide : Product  Inputs=*/  OutDataTypeStr=single
  Product : Product  OutDataTypeStr=single
  Product1 : Product  OutDataTypeStr=single
  Subtract : Sum  Inputs=+-  OutDataTypeStr=single
  Switch : Switch  Criteria=u2 > Threshold  SaturateOnIntegerOverflow=off  InputSameDT=off
  Voltage Measurement : spsVoltageMeasurementLib/Voltage Measurement  PhasorSimulation=off  OutputType=Complex  PSBequivalent=0
  - : PMIOPort  Side=Left
  + : PMIOPort  Port=2  Side=Left
  CurC_Cap : Outport
  wires:
  Add/1 -> Switch/1
  Constant3/1 -> Subtract/2
  Product/1 -> Subtract/1
  Divide/1 -> Product/2
  Constant/1 -> Add/2, Switch/3
  Subtract/1 -> Product1/1  "CurC_ADC"
  Voltage Measurement/1 -> Add/1
  Constant1/1 -> Divide/2
  Constant4/1 -> Product1/2
  Switch/1 -> Divide/1
  Constant2/1 -> Product/1
  Product1/1 -> CurC_Cap/1  "CurC_LowTerCap"
  CaptureEna/1 -> Switch/2
  connections:
  Voltage Measurement/LConn2 -- -/RConn1
  Voltage Measurement/LConn1 -- +/RConn1

== system MtrCtrl_24V/Inverter/Subsystem/Subsystem4 ==
  CaptureEna : Inport
  Add : Sum
  Constant : Constant  Value=2.5
  Constant1 : Constant  Value=5
  Constant2 : Constant  Value=4096
  Constant3 : Constant  Value=2048
  Constant4 : Constant  Value=1.221
  Divide : Product  Inputs=*/
  Product : Product
  Product1 : Product  OutDataTypeStr=single
  Subtract : Sum  Inputs=+-  OutDataTypeStr=single
  Switch : Switch  Criteria=u2 > Threshold  SaturateOnIntegerOverflow=off  InputSameDT=off
  Voltage Measurement : spsVoltageMeasurementLib/Voltage Measurement  PhasorSimulation=off  OutputType=Complex  PSBequivalent=0
  - : PMIOPort  Side=Left
  + : PMIOPort  Port=2  Side=Left
  CurC_Cap : Outport
  wires:
  CaptureEna/1 -> Switch/2
  Product1/1 -> CurC_Cap/1  "CurC_LowTerCap"
  Constant2/1 -> Product/1
  Switch/1 -> Divide/1
  Constant4/1 -> Product1/2
  Constant1/1 -> Divide/2
  Voltage Measurement/1 -> Add/1
  Subtract/1 -> Product1/1  "CurC_ADC"
  Constant/1 -> Switch/3, Add/2
  Divide/1 -> Product/2
  Product/1 -> Subtract/1
  Constant3/1 -> Subtract/2
  Add/1 -> Switch/1
  connections:
  Voltage Measurement/LConn1 -- +/RConn1
  Voltage Measurement/LConn2 -- -/RConn1

== system MtrCtrl_24V/Inverter/Subsystem/Subsystem5 ==
  CaptureEna : Inport
  Add : Sum
  Constant : Constant  Value=2.5
  Constant1 : Constant  Value=5
  Constant2 : Constant  Value=4096
  Constant3 : Constant  Value=2048
  Constant4 : Constant  Value=1.221
  Divide : Product  Inputs=*/
  Product : Product
  Product1 : Product  OutDataTypeStr=single
  Subtract : Sum  Inputs=+-  OutDataTypeStr=single
  Switch : Switch  Criteria=u2 > Threshold  SaturateOnIntegerOverflow=off  InputSameDT=off
  Voltage Measurement : spsVoltageMeasurementLib/Voltage Measurement  PhasorSimulation=off  OutputType=Complex  PSBequivalent=0
  - : PMIOPort  Side=Left
  + : PMIOPort  Port=2  Side=Left
  CurB_Cap : Outport
  wires:
  Add/1 -> Switch/1
  Constant3/1 -> Subtract/2
  Product/1 -> Subtract/1
  Divide/1 -> Product/2
  Constant/1 -> Add/2, Switch/3
  Subtract/1 -> Product1/1  "CurC_ADC"
  Voltage Measurement/1 -> Add/1
  Constant1/1 -> Divide/2
  Constant4/1 -> Product1/2
  Switch/1 -> Divide/1
  Constant2/1 -> Product/1
  Product1/1 -> CurB_Cap/1  "CurB_Cap"
  CaptureEna/1 -> Switch/2
  connections:
  Voltage Measurement/LConn2 -- -/RConn1
  Voltage Measurement/LConn1 -- +/RConn1

== system MtrCtrl_24V/Inverter/Subsystem/Subsystem6 ==
  CaptureEna : Inport
  Add : Sum
  Constant : Constant  Value=2.5
  Constant1 : Constant  Value=5
  Constant2 : Constant  Value=4096
  Constant3 : Constant  Value=2048
  Constant4 : Constant  Value=1.221
  Divide : Product  Inputs=*/
  Product : Product
  Product1 : Product  OutDataTypeStr=single
  Subtract : Sum  Inputs=+-  OutDataTypeStr=single
  Switch : Switch  Criteria=u2 > Threshold  SaturateOnIntegerOverflow=off  InputSameDT=off
  Voltage Measurement : spsVoltageMeasurementLib/Voltage Measurement  PhasorSimulation=off  OutputType=Complex  PSBequivalent=0
  - : PMIOPort  Side=Left
  + : PMIOPort  Port=2  Side=Left
  CurA_Cap : Outport
  wires:
  Add/1 -> Switch/1
  Constant3/1 -> Subtract/2
  Product/1 -> Subtract/1
  Divide/1 -> Product/2
  Constant/1 -> Add/2, Switch/3
  Subtract/1 -> Product1/1  "CurC_ADC"
  Voltage Measurement/1 -> Add/1
  Constant1/1 -> Divide/2
  Constant4/1 -> Product1/2
  Switch/1 -> Divide/1
  Constant2/1 -> Product/1
  Product1/1 -> CurA_Cap/1  "CurA_LowTerCap"
  CaptureEna/1 -> Switch/2
  connections:
  Voltage Measurement/LConn2 -- -/RConn1
  Voltage Measurement/LConn1 -- +/RConn1

== system MtrCtrl_24V/MotorModel/Subsystem/ClarkeTF ==
  Va : Inport
  Vb : Inport  Port=2
  Add : Sum  Inputs=+++
  Gain : Gain  Gain=1/sqrt(3)
  V_alpha : Outport
  V_beta : Outport  Port=2
  wires:
  Add/1 -> Gain/1
  Vb/1 -> Add/3, Add/2
  Va/1 -> V_alpha/1, Add/1
  Gain/1 -> V_beta/1

== system MtrCtrl_24V/MotorModel/Subsystem/InversePark ==
  D : Inport
  Q : Inport  Port=2
  SinTheta : Inport  Port=3
  CosTheta : Inport  Port=4
  Scope : Scope  NumInputPorts=2
  dcos : Product  RndMeth=Simplest  OutDataTypeStr=Inherit: Same as first input
  dsin : Product  RndMeth=Simplest  OutDataTypeStr=Inherit: Same as first input
  qcos : Product  RndMeth=Simplest  OutDataTypeStr=Inherit: Same as first input
  qsin : Product  RndMeth=Simplest  OutDataTypeStr=Inherit: Same as first input
  sum_alpha : Sum  Inputs=|+-  RndMeth=Simplest  OutDataTypeStr=Inherit: Same as first input
  sum_beta : Sum  Inputs=|++  RndMeth=Simplest  OutDataTypeStr=Inherit: Same as first input
  Alpha : Outport
  Beta : Outport  Port=2
  wires:
  sum_alpha/1 -> Scope/1, Alpha/1
  sum_beta/1 -> Scope/2, Beta/1
  dsin/1 -> sum_beta/2
  qcos/1 -> sum_beta/1
  CosTheta/1 -> dcos/2, qcos/2
  qsin/1 -> sum_alpha/2
  SinTheta/1 -> qsin/2, dsin/2
  Q/1 -> qcos/1, qsin/1
  dcos/1 -> sum_alpha/1
  D/1 -> dsin/1, dcos/1

== system MtrCtrl_24V/MotorModel/Subsystem/ParkTF ==
  Valpha : Inport
  Vbeta : Inport  Port=2
  SinTheta : Inport  Port=3
  CosTheta : Inport  Port=4
  Add : Sum
  Add1 : Sum  Inputs=+-
  Product{,1..3} (4 alike) : Product
  Vd : Outport
  Vq : Outport  Port=2
  wires:
  Product/1 -> Add/1
  Product1/1 -> Add/2
  Add/1 -> Vd/1
  Add1/1 -> Vq/1
  Product3/1 -> Add1/1
  Product2/1 -> Add1/2
  Valpha/1 -> Product2/1, Product/1
  SinTheta/1 -> Product2/2, Product1/2
  Vbeta/1 -> Product1/1, Product3/1
  CosTheta/1 -> Product/2, Product3/2

== system MtrCtrl_24V/MotorModel/Subsystem/Subsystem ==
  Vd : Inport
  Vq : Inport  Port=2
  we : Inport  Port=3
  Add : Sum  Inputs=+-+
  Add1 : Sum  Inputs=---+
  Constant : Constant  Value=Lq
  Constant1 : Constant  Value=Rs
  Constant2 : Constant  Value=1/Ld
  Constant3 : Constant  Value=Ld
  Constant4 : Constant  Value=Rs
  Constant5 : Constant  Value=1/Lq
  Constant6 : Constant  Value=Flux
  Discrete-Time Integrator : DiscreteIntegrator  SampleTime=-1  ICPrevOutput=DiscIntNeverNeededParam  ICPrevScaledInput=DiscIntNeverNeededParam
  Discrete-Time Integrator1 : DiscreteIntegrator  SampleTime=-1  ICPrevOutput=DiscIntNeverNeededParam  ICPrevScaledInput=DiscIntNeverNeededParam
  Product : Product  Inputs=3
  Product{1..2,4..6} (5 alike) : Product
  Product3 : Product  Inputs=3
  Scope : Scope
  Id : Outport
  Iq : Outport  Port=2
  wires:
  Discrete-Time Integrator/1 -> Scope/1, Product1/2, Product3/1, Id/1  "Id"
  Vd/1 -> Add/1
  we/1 -> Product6/2, Product3/3, Product/1
  Product5/1 -> Discrete-Time Integrator1/1
  Constant/1 -> Product/2
  Product/1 -> Add/3
  Constant1/1 -> Product1/1
  Product1/1 -> Add/2
  Add/1 -> Product2/1
  Product2/1 -> Discrete-Time Integrator/1
  Constant2/1 -> Product2/2
  Vq/1 -> Add1/4
  Product3/1 -> Add1/2
  Constant3/1 -> Product3/2
  Product4/1 -> Add1/1
  Constant4/1 -> Product4/2
  Constant5/1 -> Product5/2
  Add1/1 -> Product5/1
  Product6/1 -> Add1/3
  Constant6/1 -> Product6/1
  Discrete-Time Integrator1/1 -> Product4/1, Product/3, Iq/1  "Id"

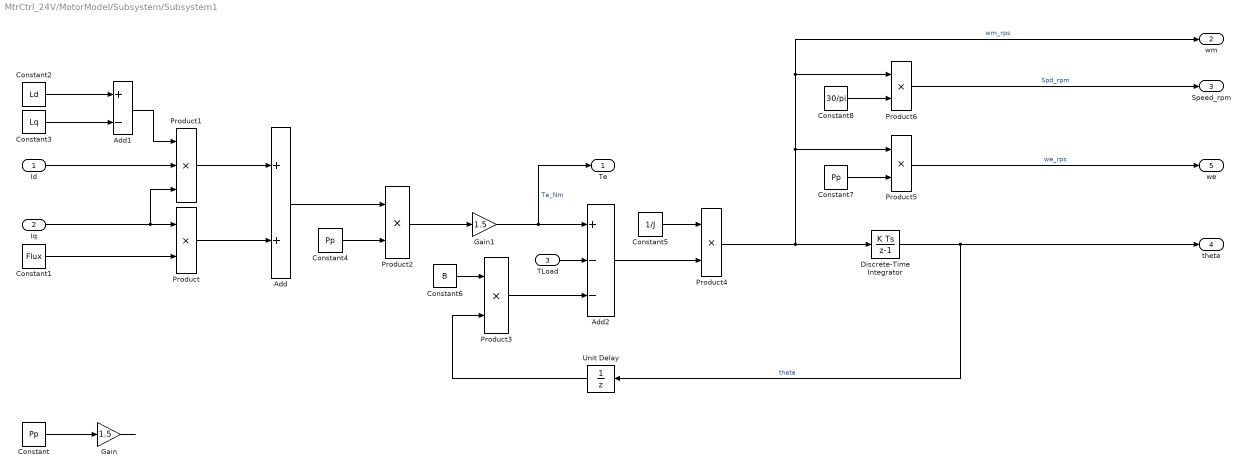
== system MtrCtrl_24V/MotorModel/Subsystem/Subsystem1 ==
  Id : Inport
  Iq : Inport  Port=2
  TLoad : Inport  Port=3
  Add : Sum
  Add1 : Sum  Inputs=+-
  Add2 : Sum  Inputs=+--
  Constant : Constant  Value=Pp
  Constant1 : Constant  Value=Flux
  Constant2 : Constant  Value=Ld
  Constant3 : Constant  Value=Lq
  Constant4 : Constant  Value=Pp
  Constant5 : Constant  Value=1/J
  Constant6 : Constant  Value=B
  Constant7 : Constant  Value=Pp
  Constant8 : Constant  Value=30/pi
  Discrete-Time Integrator : DiscreteIntegrator  SampleTime=-1  ICPrevOutput=DiscIntNeverNeededParam  ICPrevScaledInput=DiscIntNeverNeededParam
  Gain : Gain  Gain=1.5
  Gain1 : Gain  Gain=1.5
  Product{,2..6} (6 alike) : Product
  Product1 : Product  Inputs=3
  Unit Delay : UnitDelay  SampleTime=-1  HasFrameUpgradeWarning=on
  Te : Outport
  wm : Outport  Port=2
  Speed_rpm : Outport  Port=3
  theta : Outport  Port=4
  we : Outport  Port=5
  wires:
  Iq/1 -> Product1/3, Product/1
  Constant/1 -> Gain/1
  Id/1 -> Product1/2
  Constant1/1 -> Product/2
  Gain/1 -> ?
  Product/1 -> Add/2
  Add1/1 -> Product1/1
  Constant2/1 -> Add1/1
  Constant3/1 -> Add1/2
  Product1/1 -> Add/1
  Add/1 -> Product2/1
  Constant4/1 -> Product2/2
  Product2/1 -> Gain1/1
  Gain1/1 -> Add2/1, Te/1  "Te_Nm"
  TLoad/1 -> Add2/2
  Constant7/1 -> Product5/2
  Product5/1 -> we/1  "we_rps"
  Product6/1 -> Speed_rpm/1  "Spd_rpm"
  Constant8/1 -> Product6/2
  Discrete-Time Integrator/1 -> theta/1, Unit Delay/1  "theta"
  Add2/1 -> Product4/2
  Constant5/1 -> Product4/1
  Product4/1 -> Discrete-Time Integrator/1, Product5/1, Product6/1, wm/1  "wm_rps"
  Unit Delay/1 -> Product3/2
  Product3/1 -> Add2/3
  Constant6/1 -> Product3/1

== system MtrCtrl_24V/MotorModel/Subsystem/Subsystem2 ==
  Theta_In : Inport
  Theta_Mtr : Inport  Port=2
  Add : Sum  Inputs=+-
  Constant : Constant  Value=2*pi
  Constant1 : Constant  Value=Pp
  Constant2 : Constant  Value=PosnSelector
  Divide : Product  Inputs=*/  OutDataTypeStr=uint16
  Product : Product
  Product1 : Product
  Scope1 : Scope  NumInputPorts=2
  SinCos : Trigonometry  Operator=sincos
  Switch : Switch  Criteria=u2 > Threshold  SaturateOnIntegerOverflow=off  InputSameDT=off
  SinTheta : Outport
  CoTheta : Outport  Port=2
  wires:
  Theta_In/1 -> Scope1/1, Switch/1
  Constant/1 -> Product1/2, Divide/2
  Divide/1 -> Product1/1
  Add/1 -> SinCos/1
  Product1/1 -> Add/2
  SinCos/1 -> SinTheta/1
  SinCos/2 -> CoTheta/1
  Theta_Mtr/1 -> Scope1/2, Switch/3
  Constant1/1 -> Product/1
  Product/1 -> Add/1, Divide/1
  Switch/1 -> Product/2
  Constant2/1 -> Switch/2

== system MtrCtrl_24V/MotorModel/Subsystem/Subsystem3 ==
  Alpha : Inport
  Beta : Inport  Port=2
  Add : Sum  Inputs=-+
  Add1 : Sum  Inputs=--
  one_by_two : Gain  Gain=1/2  RndMeth=Simplest  OutDataTypeStr=Inherit: Same as input
  sqrt3_by_two : Gain  Gain=sqrt(3)/2  RndMeth=Simplest  OutDataTypeStr=Inherit: Same as input
  CurA : Outport  VectorParamsAs1DForOutWhenUnconnected=off
  CurB : Outport  Port=2  VectorParamsAs1DForOutWhenUnconnected=off
  CurC : Outport  Port=3  VectorParamsAs1DForOutWhenUnconnected=off
  wires:
  sqrt3_by_two/1 -> Add/2, Add1/2
  Add1/1 -> CurC/1
  one_by_two/1 -> Add/1, Add1/1
  Alpha/1 -> CurA/1, one_by_two/1
  Beta/1 -> sqrt3_by_two/1
  Add/1 -> CurB/1

== system MtrCtrl_24V/CurLpCtrl/SVPWM/Overmodulation/Subsystem2 ==
  Ts : Inport  OutDataTypeStr=fixdt(0,32,32)
  Tx : Inport  Port=2  OutDataTypeStr=fixdt(0,32,30)
  Ty : Inport  Port=3  OutDataTypeStr=fixdt(0,32,30)
  Add : Sum  OutDataTypeStr=fixdt(0,32,32)
  Add1 : Sum  Inputs=-+  OutDataTypeStr=fixdt(1,32,4)
  Add2 : Sum  Inputs=+--  OutDataTypeStr=fixdt(0,32,32)
  Compare To Constant : simulink/Logic and Bit Operations/Compare To Constant  relop=>=  const=0  OutDataTypeStr=boolean
  Divide : Product  Inputs=*/  OutDataTypeStr=fixdt(0,32,20)
  Product : Product  OutDataTypeStr=fixdt(0,32,32)
  Switch : Switch  Criteria=u2 > Threshold  OutDataTypeStr=fixdt(0,32,33)  SaturateOnIntegerOverflow=off  InputSameDT=off
  Switch1 : Switch  Criteria=u2 > Threshold  OutDataTypeStr=fixdt(0,32,33)  SaturateOnIntegerOverflow=off  InputSameDT=off
  Tx_o : Outport
  Ty_o : Outport  Port=2
  wires:
  Compare To Constant/1 -> Switch/2, Switch1/2
  Add1/1 -> Switch1/3  "Ty'"
  Switch/1 -> Tx_o/1
  Switch1/1 -> Ty_o/1
  Add2/1 -> Compare To Constant/1
  Product/1 -> Add1/1, Switch/3  "Tx'"
  Divide/1 -> Product/1
  Tx/1 -> Add2/2, Add/1, Switch/1, Product/2
  Ts/1 -> Divide/1, Add2/1, Add1/2
  Add/1 -> Divide/2
  Ty/1 -> Add/2, Switch1/1, Add2/3
